simulink model "MCuC_Model"  (R2023b)
settings: Solver=ode8  StartTime=0.0  StopTime=10.0  FixedStep=.0001  RelTol=1e-3
libraries: msbUtilities x1
settings Model: Creator=mjmag  LastModifiedBy=mjmag

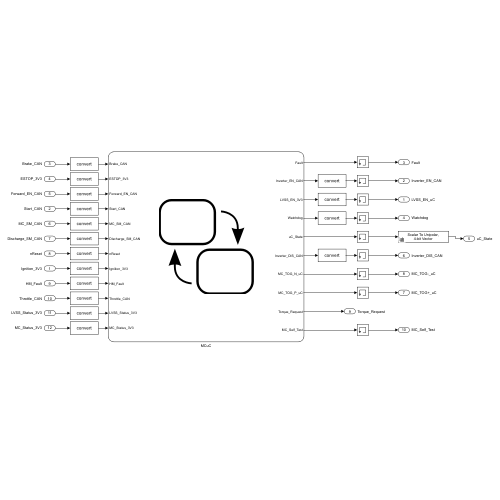
[thumbnail: Simulink's stored preview of the top-level diagram]
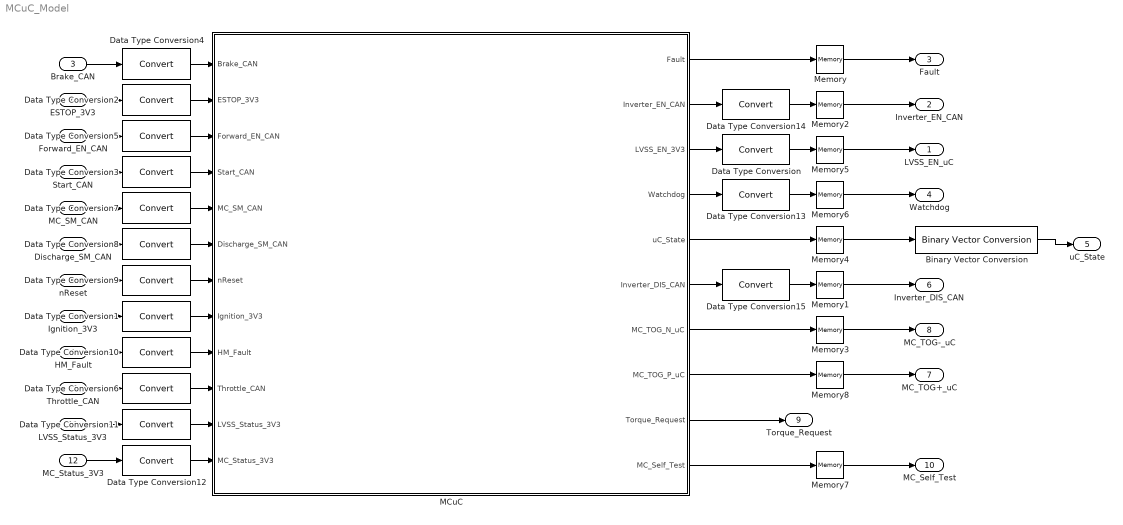
== system MCuC_Model ==
  Ignition_3V3 : Inport  OutDataTypeStr=boolean
  Start_CAN : Inport  Port=2  OutDataTypeStr=boolean
  Brake_CAN : Inport  Port=3  OutDataTypeStr=int16
  ESTOP_3V3 : Inport  Port=4  OutDataTypeStr=boolean
  Forward_EN_CAN : Inport  Port=5  OutDataTypeStr=boolean
  MC_SM_CAN : Inport  Port=6  OutDataTypeStr=uint8
  Discharge_SM_CAN : Inport  Port=7  OutDataTypeStr=uint8
  nReset : Inport  Port=8  OutDataTypeStr=boolean
  HM_Fault : Inport  Port=9  OutDataTypeStr=boolean
  Throttle_CAN : Inport  Port=10  OutDataTypeStr=int16
  LVSS_Status_3V3 : Inport  Port=11  OutDataTypeStr=boolean
  MC_Status_3V3 : Inport  Port=12  OutDataTypeStr=boolean
  Binary Vector Conversion : msbUtilities/Binary Vector Conversion  LabelModeActiveChoice=To Unipolar  Convert=Scalar to binary-coded vector  Encoding=Unipolar (magnitude)  InputLength=8  InputReverse=LSB at index 1  OutputLength=4  OutputReverse=LSB at index 1  DataType=double
  Data Type Conversion{,1..15} (16 alike) : DataTypeConversion  SaturateOnIntegerOverflow=off  RndMeth=Floor
  MCuC : Stateflow chart  TreatAsAtomicUnit=on
      settings: PortSchema="{\"entries\":[{\"content\":{\"sides\":[{\"content\":{\"connectorIds\":[\"In1\",\"In2\",\"In3\",\"In5\",\"In6\",\"In7\",\"In8\",\"In4\",\"In9\",\"In10\",\"In11\",\"In12\"]},\"type\":\"ConnectorPlacement.EquallySpacedRectSide\",\"uuid\":\"d1510c73-f1c7-4e03-bb6c-bda7856f993e\"},{\"content\":{\"connectorIds\":[\"Out1\",\"Out2\",\"Out3\",\"Out4\",\"Out5\",\"Out6\",\"Out7\",\"Out8\",\"Out9\",\"Out10\"],\"side\":\"RIGHT\"},\"type\":\"ConnectorPlacement.EquallySpacedRectSide\",\"uuid\":\"1a7878c4-a817-4ca0-b21c-0429e82bb9d7\"},{\"content\":{\"side\":\"TOP\"},\"type\":\"ConnectorPlacement.EquallySpacedRectSide\",\"uuid\":\"ed9f2701-7044-4bb4-9c0b-b9cf9840e69e\"}]},\"type\":\"ConnectorPlacement.EquallySpacedConnector\",\"uuid\":\"4ceb8e7d-629c-4438-88a9-aa3016537644\"}],\"packageUris\":[\"http://schema.mathworks.com/mf0/Connector/R2020b\"],\"version\":\"1.0\"}"
  Memory{,1..8} (9 alike) : Memory
  LVSS_EN_uC : Outport  OutDataTypeStr=boolean
  Inverter_EN_CAN : Outport  Port=2
  Fault : Outport  Port=3
  Watchdog : Outport  Port=4  OutDataTypeStr=boolean
  uC_State : Outport  Port=5  OutDataTypeStr=boolean
  Inverter_DIS_CAN : Outport  Port=6
  MC_TOG+_uC : Outport  Port=7
  MC_TOG-_uC : Outport  Port=8
  Torque_Request : Outport  Port=9
  MC_Self_Test : Outport  Port=10
  wires:
  Forward_EN_CAN/1 -> Data Type Conversion5/1
  Ignition_3V3/1 -> Data Type Conversion1/1
  MCuC/5(uC_State) -> Memory4/1
  MCuC/3(LVSS_EN_3V3) -> Data Type Conversion/1
  Discharge_SM_CAN/1 -> Data Type Conversion8/1
  Start_CAN/1 -> Data Type Conversion3/1
  ESTOP_3V3/1 -> Data Type Conversion2/1
  Memory4/1 -> Binary Vector Conversion/1
  HM_Fault/1 -> Data Type Conversion10/1
  LVSS_Status_3V3/1 -> Data Type Conversion11/1
  MCuC/1(Fault) -> Memory/1
  MCuC/10(MC_Self_Test) -> Memory7/1
  MCuC/4(Watchdog) -> Data Type Conversion13/1
  Throttle_CAN/1 -> Data Type Conversion6/1
  Binary Vector Conversion/1 -> uC_State/1
  Memory7/1 -> MC_Self_Test/1
  Data Type Conversion/1 -> Memory5/1
  Memory1/1 -> Inverter_DIS_CAN/1
  MCuC/2(Inverter_EN_CAN) -> Data Type Conversion14/1
  MC_SM_CAN/1 -> Data Type Conversion7/1
  Memory5/1 -> LVSS_EN_uC/1
  MC_Status_3V3/1 -> Data Type Conversion12/1
  nReset/1 -> Data Type Conversion9/1
  MCuC/7(MC_TOG_N_uC) -> Memory3/1
  Memory2/1 -> Inverter_EN_CAN/1
  Memory/1 -> Fault/1
  MCuC/9(Torque_Request) -> Torque_Request/1
  Memory3/1 -> MC_TOG-_uC/1
  Memory8/1 -> MC_TOG+_uC/1
  Memory6/1 -> Watchdog/1
  MCuC/6(Inverter_DIS_CAN) -> Data Type Conversion15/1
  MCuC/8(MC_TOG_P_uC) -> Memory8/1
  Brake_CAN/1 -> Data Type Conversion4/1
  Data Type Conversion1/1 -> MCuC/4(Ignition_3V3)
  Data Type Conversion2/1 -> MCuC/2(ESTOP_3V3)
  Data Type Conversion3/1 -> MCuC/5(Start_CAN)
  Data Type Conversion4/1 -> MCuC/1(Brake_CAN)
  Data Type Conversion5/1 -> MCuC/3(Forward_EN_CAN)
  Data Type Conversion6/1 -> MCuC/10(Throttle_CAN)
  Data Type Conversion7/1 -> MCuC/6(MC_SM_CAN)
  Data Type Conversion8/1 -> MCuC/7(Discharge_SM_CAN)
  Data Type Conversion9/1 -> MCuC/8(nReset)
  Data Type Conversion10/1 -> MCuC/9(HM_Fault)
  Data Type Conversion11/1 -> MCuC/11(LVSS_Status_3V3)
  Data Type Conversion12/1 -> MCuC/12(MC_Status_3V3)
  Data Type Conversion13/1 -> Memory6/1
  Data Type Conversion14/1 -> Memory2/1
  Data Type Conversion15/1 -> Memory1/1

== stateflow chart MCuC_Model/MCuC ==
  state MCuC
    state MCuC_Logic [parallel]
      settings: executionOrder=1
      state MC_Off
        entry:
        LVSS_EN_3V3 = 0;
        uC_State = 0;
        uncharged = 1;
        Inverter_EN_CAN = 0;
      state LVSS_MC_Shutdown
        entry:
        uC_State = 10;
        LVSS_EN_3V3 = 0;
        Inverter_DIS_CAN = 0;
        MC_TOG_P_uC = 0;
        MC_TOG_N_uC = 1;
        exit:
        MC_TOG_P_uC = 0;
        MC_TOG_N_uC = 0;
      state MC_Discharging
        entry:
        uC_State = 5;
      state ESTOP
        entry:
        uC_State = 7;
        LVSS_EN_3V3 = 0;
        ESTOP_activated = 0;
      state Fault_Ignit_H
      state LVSS_MC_Startup
        entry:
        uncharged = 0;
        uC_State = 10;
        LVSS_EN_3V3 = 1;
        MC_TOG_P_uC = 1;
        MC_TOG_N_uC = 0;
        exit:
        MC_TOG_P_uC = 0;
        MC_TOG_N_uC = 0;
      state Fault
        entry:
        uC_State = 6;
        Fault_Activated = 0;
        Fault = 1;
        exit:
        Fault = 0;
      state Contactor_Open
        entry:
        Inverter_EN_CAN = 0;
        Inverter_DIS_CAN = 1;
        uC_State = 4;
      state MC_Init
        entry:
        uC_State = 1;
      state Preset
        entry:
        uC_State = 8;
        state MC_ST
          entry:
          MC_Self_Test = 1
          state MC_EN_ON
            entry:
            MC_TOG_P_uC = 1;
            MC_TOG_N_uC = 0;
          state MC_EN_OFF
            entry:
            MC_TOG_P_uC = 0;
            MC_TOG_N_uC = 1;
          (default) -> MC_EN_ON
          MC_EN_ON -> MC_EN_OFF : [MC_Status_3V3 == 1]
        (default) -> MC_ST
      state MC_Active
        entry:
        Inverter_EN_CAN = 1;
        uC_State = 3;
        Torque_Request = 0;
        during:
        Torque_Request = Throttle_CAN;
        exit:
        Torque_Request = 0;
      state Contactor_Closed
        entry:
        uC_State = 2;
        Inverter_EN_CAN = 0;
      LVSS_MC_Shutdown -> MC_Off : [MC_Status_3V3 == 0 && LVSS_Status_3V3 == 0]
      Fault_Ignit_H -> MC_Off : [Ignition_3V3 == 0]
      MC_Discharging -> LVSS_MC_Shutdown : [Discharge_SM_CAN == 4]
      MCuC_Logic -> ESTOP [order 3] : [ESTOP_3V3 == 1 && uncharged == 1 && nReset == 1 && uC_State ~= 8]
      ESTOP -> MC_Off : [ESTOP_3V3 == 0]
      Preset -> MC_Off : [MC_Status_3V3 == 0 && Ignition_3V3 == 0 && LVSS_Status_3V3 == 0]
          | {MC_Self_Test = 0}
      MC_Off -> LVSS_MC_Startup : [Ignition_3V3 == 1]
      Contactor_Open -> MC_Discharging : [Discharge_SM_CAN ~= 0]
      Fault -> Fault_Ignit_H : [MC_Status_3V3 == 0 && Ignition_3V3 == 1]
      MCuC_Logic -> Fault [order 4] : [HM_Fault == 1 && uncharged == 1 && uC_State ~= 8 && nReset == 1]
      LVSS_MC_Startup -> MC_Init : [MC_Status_3V3 == 1 && LVSS_Status_3V3 == 1]
      (default) -> Preset
      MCuC_Logic -> Contactor_Open [order 1] : [HM_Fault == 1 && Ignition_3V3 == 1 && uncharged == 0 && Fault_Activated == 0]{Fault_Activated = 1}
      MCuC_Logic -> Contactor_Open [order 2] : [ESTOP_3V3 == 1 && uncharged == 0 && ESTOP_activated == 0]{ESTOP_activated = 1}
      MCuC_Logic -> Preset [order 5] : [nReset == 0]
      MC_Init -> Contactor_Open [order 1] : [Ignition_3V3 == 0]
      Contactor_Closed -> Contactor_Open [order 2] : [Ignition_3V3 == 0]
      MC_Active -> Contactor_Open [order 2] : [Ignition_3V3 == 0]
      MC_Init -> Contactor_Closed [order 2] : [MC_SM_CAN == 5]
      Contactor_Closed -> MC_Active [order 1] : [Start_CAN == 1 && Forward_EN_CAN == 1 && Brake_CAN == 1 && Throttle_CAN == 0]
      MC_Active -> Contactor_Closed [order 1] : [Forward_EN_CAN == 0]
    state Watchdog [parallel]
      settings: executionOrder=2
      state WD0
        entry:
        Watchdog = 0;
      state WD1
        entry:
        Watchdog = 1;
      (default) -> WD0
      WD0 -> WD1 : after(.5, sec)
      WD1 -> WD0 : after(.5, sec)
  data: Fault output =0; Brake_CAN input; ESTOP_3V3 input; Forward_EN_CAN input; Ignition_3V3 input; Start_CAN input; MC_SM_CAN input; Inverter_EN_CAN output =0; LVSS_EN_3V3 output =0; Discharge_SM_CAN input; nReset input; Watchdog output =0; uC_State output =0; uncharged local =1; ESTOP_activated local =0; HM_Fault input; Throttle_CAN input; Inverter_DIS_CAN output =0; MC_TOG_N_uC output =0; MC_TOG_P_uC output =0; LVSS_Status_3V3 input; MC_Status_3V3 input; Torque_Request output =0; Fault_Activated local =0; MC_Self_Test output
